simulink model "Integrator_verif"  (Simulink 7.2)
settings: Solver=ode45  StartTime=0.0  StopTime=10.0  RelTol=1e-3
undefined symbols (not defined in the file): integrator_sample
settings Model: Creator=Romain  LastModifiedBy=Romain
settings OptimizationCC: ExpressionDepthLimit=128
settings DebuggingCC: SolverPrmCheckMsg=none  FcnCallInpInsideContextMsg=Enable All  StateNameClashWarn=none  StrictBusMsg=ErrorLevel1
settings CodeAppCC: CustomSymbolStrType=$N$R$M_T
settings GRTTargetCC: TargetFunctionLibrary=C89/C90 (ANSI)

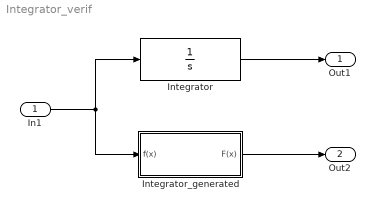
== system Integrator_verif ==
  In1 : Inport  OutDataTypeStr=double  DataType=double
  Integrator : Integrator
  Integrator_generated : Subsystem  TreatAsAtomicUnit=on
  Out1 : Outport
  Out2 : Outport  Port=2
  wires:
  In1/1 -> Integrator_generated/1(f(x)), Integrator/1
  Integrator/1 -> Out1/1
  Integrator_generated/1(F(x)) -> Out2/1

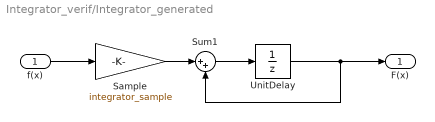
== system Integrator_verif/Integrator_generated ==
  f(x) : Inport
  Sample : Gain  Gain=integrator_sample
  Sum1 : Sum  RequirementInfo={} %GIDa_282a7a86_0b36_4049_b4f9_00baf84ce7ac  Inputs=|++
  UnitDelay : UnitDelay  SampleTime=integrator_sample
  F(x) : Outport  RequirementInfo={} %GIDa_73899e70_f018_48e1_9477_d76a1516d37e
  wires:
  f(x)/1 -> Sample/1
  UnitDelay/1 -> Sum1/2, F(x)/1
  Sum1/1 -> UnitDelay/1
  Sample/1 -> Sum1/1
